simulink model "RobotTrajectoryTracking"  (R2023a)
settings: Solver=ode45  StartTime=0.0  StopTime=10  RelTol=1e-3
libraries: slpidlib x4, nesl_utility x1
settings Model: Creator=kming  LastModifiedBy=kming

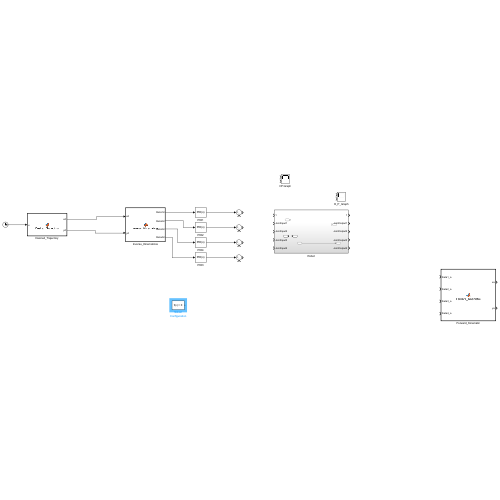
[thumbnail: Simulink's stored preview of the top-level diagram]
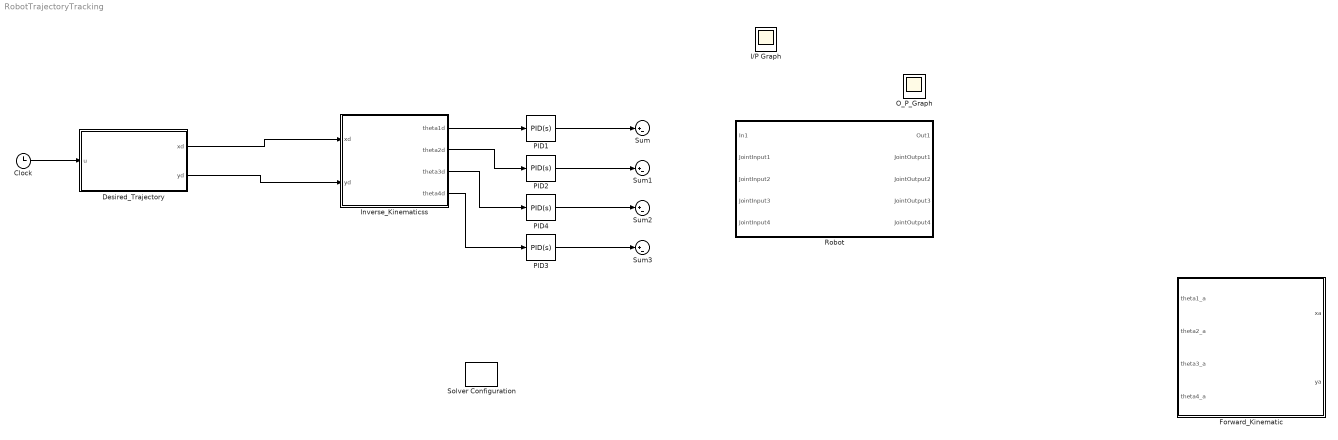
== system RobotTrajectoryTracking ==
  Clock : Clock
  Desired_Trajectory : MATLAB Function  TreatAsAtomicUnit=on
  Forward_Kinematic : MATLAB Function  TreatAsAtomicUnit=on
  I/P Graph : Scope  NumInputPorts=2
  Inverse_Kinematicss : MATLAB Function  TreatAsAtomicUnit=on
  O_P_Graph : Scope  NumInputPorts=2
  PID{1..4} (4 alike) : slpidlib/PID Controller  Controller=PID  Form=Parallel  TimeDomain=Continuous-time  UseExternalTs=off  SampleTime=-1  IntegratorMethod=Forward Euler  FilterMethod=Forward Euler  ControllerParametersSource=internal  P=10  I=1  UseKiTs=off  D=0.1  N=100  UseFilter=on  TunerSelectOption=Transfer Function Based (PID Tuner App)  InitialConditionSource=internal  InitialConditionForIntegrator=0  InitialConditionForFilter=0  DifferentiatorICPrevScaledInput=0  ExternalReset=none  TrackingMode=off  Kt=1  LimitOutput=off  SatLimitsSource=internal  UpperSaturationLimit=inf  LowerSaturationLimit=-inf  LinearizeAsGain=on  AntiWindupMode=none  Kb=1  LimitIntegrator=off  UpperIntegratorSaturationLimit=inf  LowerIntegratorSaturationLimit=-inf  POutMin=[]  POutMax=[]  IOutMin=[]  IOutMax=[]  DOutMin=[]  DOutMax=[]  NOutMin=[]  NOutMax=[]  SumOutMin=[]  SumOutMax=[]  SaturationOutMin=[]  SaturationOutMax=[]  PParamMin=[]  PParamMax=[]  IParamMin=[]  IParamMax=[]  DParamMin=[]  DParamMax=[]  NParamMin=[]  NParamMax=[]  KbParamMin=[]  KbParamMax=[]  KtParamMin=[]  KtParamMax=[]  KbOutMin=[]  KbOutMax=[]  KtOutMin=[]  KtOutMax=[]  IntegratorOutMin=[]  IntegratorOutMax=[]  FilterOutMin=[]  FilterOutMax=[]  SumI1OutMin=[]  SumI1OutMax=[]  SumI2OutMin=[]  SumI2OutMax=[]  SumI3OutMin=[]  SumI3OutMax=[]  SumI4OutMin=[]  SumI4OutMax=[]  SumDOutMin=[]  SumDOutMax=[]  DifferentiatorOutMin=[]  DifferentiatorOutMax=[]  FilterDiffOutCoefMin=[]  FilterDiffOutCoefMax=[]  ReciprocalOutMin=[]  ReciprocalOutMax=[]  SumDenOutMin=[]  SumDenOutMax=[]  SumNumOutMin=[]  SumNumOutMax=[]  DivideOutMin=[]  DivideOutMax=[]  UdiffTsProdOutMin=[]  UdiffTsProdOutMax=[]  NTsProdOutMin=[]  NTsProdOutMax=[]  UintegralTsProdOutMin=[]  UintegralTsProdOutMax=[]  UngainTsProdOutMin=[]  UngainTsProdOutMax=[]  ClampingZeroOutDataTypeStr=Inherit: Inherit via back propagation  ClampingZeroOutMin=[]  ClampingZeroOutMax=[]  FilterDenConstantOutDataTypeStr=Inherit: Inherit via back propagation  FilterDenConstantOutMin=[]  FilterDenConstantOutMax=[]  PCopyOutDataTypeStr=Inherit: Inherit via back propagation  PCopyOutMin=[]  PCopyOutMax=[]  NCopyOutDataTypeStr=Inherit: Inherit via back propagation  NCopyOutMin=[]  NCopyOutMax=[]  IntegratorContinuousStateAttributes=''  IntegratorStateMustResolveToSignalObject=off  IntegratorRTWStateStorageClass=Auto  FilterContinuousStateAttributes=''  FilterStateMustResolveToSignalObject=off  FilterRTWStateStorageClass=Auto  ParallelPVariant=InternalParameters  IdealPVariant=Disabled  IVariant=InternalParameters  DVariant=InternalParameters  IntegratorVariant=Continuous  SatVariant=Disabled  AWVariant=Passthrough  PCopyVariant=Disabled  TRVariant=Disabled  FdbkBlocksVariant=Forward  IdealPFdbkVariant=Disabled  SatFdbkVariant=Disabled  DerivativeFilterVariant=ContFilter  NVariant=InternalParameters  NCopyVariant=Disabled  FilterICVariant=InternalICsFilter  IntegratorICVariant=InternalICs  ExternalResetVariant=Disabled  TRSumVariant=Passthrough  SumFdbkVariant=Disabled  SumVariant=Sum_PID  TsampFilterVariant=InternalTs  TsampNgainVariant=Passthrough  TsampIntegralVariant=Disabled_SignalSpec  ExternalSaturationOutDataTypeStr=Inherit: Same as second input
  Robot : Subsystem
  Solver Configuration : nesl_utility/Solver Configuration  PhysicalDomain=network_engine_domain  SubClassName=solver  LeftPortType=input  RightPortType=generic  Tones=[]  Harmonics=[]  SimulateNoise=off  Profile=off  UseLocalSampling=off  EnableSwitchedLinearOptims=on  FrequencyDomain=off  UseCCode=off  RelTol=0.001  AbsTol=0.001  MinStep=1e-09  ToWorkspace=off  RevertToSquareIcSolve=off  NumHomotopyIterations=100  PhasorMode=off  PhasorModeNumHarmonics=1  ConsistencySolver=NEWTON_XTOL_AFTER_FTOL  IndexReductionMethod=DerivativeReplacement  DoDC=off  ResidualTolerance=1e-09  ConsistencyTolSource=GLOBAL  ConsistencyAbsTol=0.001  ConsistencyRelTol=0.001  ConsistencyTolFactor=0.001  UseLocalSolver=off  LocalSolverChoice=NE_BACKWARD_EULER_ADVANCER  ResolveIndetEquations=on  FunctionEvalNumThread=1  LocalSolverSampleTime=0.001  DoFixedCost=off  MaxNonlinIter=3  MaxModeIter=2  ComputeImpulses=off  ImpulseIterations=2  LinearAlgebra=auto  LinearAlgebraNumThread=0  EquationFormulation=NE_TIME_EF  DelaysMemoryBudget=1024  AutomaticFiltering=on  FilteringTimeConstant=0.001  PartitionStorageMethod=AS_NEEDED  PartitionMemoryBudget=1024  PartitionMethod=ROBUST
  Sum{,1..3} (4 alike) : Sum  Inputs=|+-
  wires:
  Desired_Trajectory/1(xd) -> Inverse_Kinematicss/1(xd)
  Inverse_Kinematicss/1(theta1d) -> PID1/1
  Inverse_Kinematicss/2(theta2d) -> PID2/1
  Inverse_Kinematicss/3(theta3d) -> PID4/1
  Inverse_Kinematicss/4(theta4d) -> PID3/1
  Desired_Trajectory/2(yd) -> Inverse_Kinematicss/2(yd)
  Clock/1 -> Desired_Trajectory/1(u)
  PID1/1 -> Sum/1
  PID2/1 -> Sum1/1
  PID3/1 -> Sum3/1
  PID4/1 -> Sum2/1

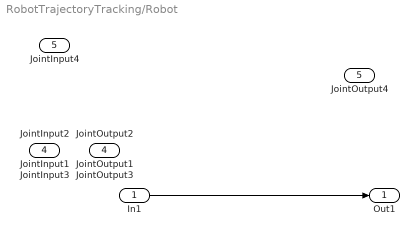
== system RobotTrajectoryTracking/Robot ==
  In1 : Inport
  JointInput1 : Inport  Port=2
  JointInput2 : Inport  Port=3
  JointInput3 : Inport  Port=4
  JointInput4 : Inport  Port=5
  Out1 : Outport
  JointOutput1 : Outport  Port=2
  JointOutput2 : Outport  Port=3
  JointOutput3 : Outport  Port=4
  JointOutput4 : Outport  Port=5
  wires:
  In1/1 -> Out1/1

== matlab function RobotTrajectoryTracking/Inverse_Kinematicss ==
  data: xd input; theta1d output; yd input; theta2d output; theta3d output; theta4d output
function [theta1d, theta2d, theta3d, theta4d] = Inverse_Kinematicss(xd, yd)
    l1 = 1;
    l2 = 2;
    l3 = 1.5;
    l4 = 1;

    % theta2d 계산
    theta2d = acos((xd^2 + yd^2 - l1^2 - l2^2) / (2 * l1 * l2));

    % theta1d 계산
    temp = (l1 + l2 * cos(theta2d));
    theta1d = atan2(yd, xd) - atan2((l2 * sin(theta2d)), temp);

    % 중간 계산값
    x = temp * cos(theta1d);
    y = temp * sin(theta1d);
    z = yd - l2 * sin(theta2d);

    % theta4d 계산
    theta4d = acos((x^2 + y^2 + z^2 - l3^2 - l4^2) / (2 * l3 * l4));

    % theta3d 계산
    num = l3^2 + l4^2 - (x^2 + y^2 + z^2);
    denom = 2 * l3 * l4;
    a = sqrt(x^2 + y^2);
    p = (num / denom)^2;
    b = sqrt(p - 1);
    theta3d = atan2(z, a) - atan2(b, num / denom);
end

== matlab function RobotTrajectoryTracking/Desired_Trajectory ==
  data: u input; xd output; yd output
function [xd, yd] = Desired_Trajectory(u)
    xd = 1 + 0.5 * sin((2 * pi / 5) * u + pi / 2);
    yd = 1 + 0.5 * cos((2 * pi / 5) * u + pi / 2);
end

== matlab function RobotTrajectoryTracking/Forward_Kinematic ==
  data: theta1_a input; xa output; theta2_a input; theta3_a input; theta4_a input; ya output
function [xa, ya] = Forward_Kinematic(theta1_a, theta2_a, theta3_a, theta4_a)
    l1 = 1;
    l2 = 1;
    l3 = 1.5;
    l4 = 1;

    xa = l1 * cos(theta1_a) + l2 * cos(theta1_a + theta2_a) + ...
         l3 * cos(theta1_a + theta2_a + theta3_a) + ...
         l4 * cos(theta1_a + theta2_a + theta3_a + theta4_a);

    ya = l1 * sin(theta1_a) + l2 * sin(theta1_a + theta2_a) + ...
         l3 * sin(theta1_a + theta2_a + theta3_a) + ...
         l4 * sin(theta1_a + theta2_a + theta3_a + theta4_a);
end
